simulink model "solarmonitor_systemblock"  (R2019b)
settings: Solver=FixedStepAuto  StartTime=0.0  StopTime=Inf  RelTol=1e-3  EnableMultiTasking=on
settings Model: Creator=shogo  LastModifiedBy=shogo
settings SolverCC: PositivePriorityOrder=on
settings OptimizationCC: EnhancedBackFolding=on  PassReuseOutputArgsAs=Individual arguments  ZeroExternalMemoryAtStartup=off  ZeroInternalMemoryAtStartup=off  MaxStackSize=64  OptimizeBlockOrder=speed  DifferentSizesBufferReuse=on  OptimizationCustomize=off  EfficientTunableParamExpr=on
settings DebuggingCC: ParameterTunabilityLossMsg=error
settings HardwareCC: ProdBitPerPointer=32  ProdBitPerSizeT=32  ProdBitPerPtrDiffT=32  ProdLargestAtomicInteger=Long  ProdLargestAtomicFloat=Double  ProdWordSize=32  ProdLongLongMode=on  ProdHWDeviceType=ARM Compatible->ARM Cortex  UseEmbeddedCoderFeatures=off  UseSimulinkCoderFeatures=off
settings RTWCC: SystemTargetFile=ert.tlc  HardwareBoard=Raspberry Pi  TLCOptions="-aInlineSetEventsForThisBaseRateFcn=TLC_FALSE -aSuppressMultiTaskScheduler=TLC_FALSE  -aRateBasedStepFcn=0"  TemplateMakefile=ert_default_tmf  RTWVerbose=off  Toolchain=GNU GCC Raspberry Pi  BuildConfiguration=Faster Runs  IncludeHyperlinkInReport=on
settings CodeAppCC: ForceParamTrailComments=on  OperatorAnnotations=on  SimulinkDataObjDesc=on  SFDataObjDesc=on  MangleLength=10  InsertBlockDesc=on
settings ERTTargetCC: TargetLangStandard=C99 (ISO)  SupportNonInlinedSFcns=on  SupportVariableSizeSignals=on  ExtMode=on  ExtModeTransport=2  ExtModeStaticAlloc=on  ExtModeMexFile=ext_xcp  ExtModeMexArgs='192.168.11.21' 0 17725  ExtModeIntrfLevel=Level2 - Open  ERTSrcFileBannerTemplate=codertarget_code_template.cgt  ERTHdrFileBannerTemplate=codertarget_code_template.cgt  ERTDataSrcFileTemplate=codertarget_code_template.cgt  ERTDataHdrFileTemplate=codertarget_code_template.cgt

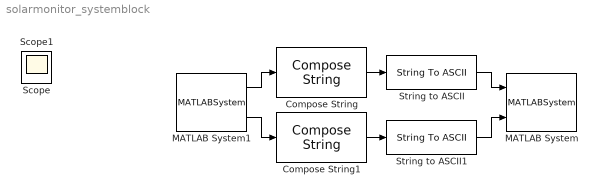
== system solarmonitor_systemblock ==
  Compose String : ComposeString  Format="\"% 7.3fV\""
  Compose String1 : ComposeString  Format="\"% 7.3fA\""
  MATLAB System : MATLABSystem  System=Aqm0802
      mask Type: Aqm0802
      mask Display:
      | disp('AQM0802');
      | port_label('input',1,'line1');
      | port_label('input',2,'line2');
  MATLAB System1 : MATLABSystem  System=Ina226  SampleTime=0.1
      mask Type: Ina226
      mask Display:
      | disp('INA226');
      | port_label('output',1,'v');
      | port_label('output',2,'c');
  String to ASCII : StringToASCII  OutputVectorSize=32
  String to ASCII1 : StringToASCII  OutputVectorSize=32
  Scope : Scope
  Scope1 : Scope
  wires:
  MATLAB System1/2 -> Compose String1/1
  String to ASCII1/1 -> MATLAB System/2
  MATLAB System1/1 -> Compose String/1
  String to ASCII/1 -> MATLAB System/1
  Compose String/1 -> String to ASCII/1
  Compose String1/1 -> String to ASCII1/1
